simulink model "mc_sevcong4s10"  (R2025a)
settings: Solver=FixedStepAuto  StartTime=0.0  StopTime=10.0  FixedStep=0.05  RelTol=1e-3
settings Model: Creator=adam  LastModifiedBy=adam

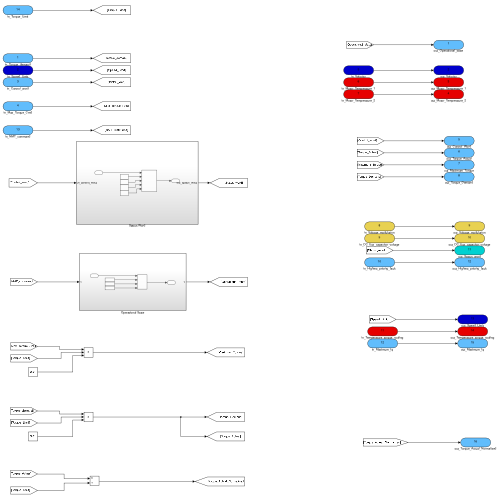
[thumbnail: Simulink's stored preview of the top-level diagram]
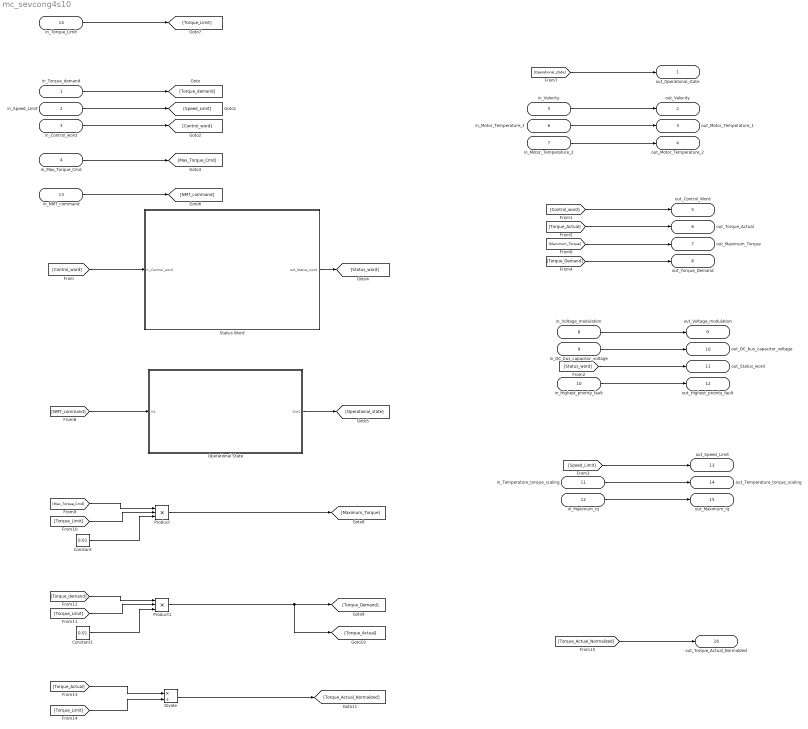
== system mc_sevcong4s10 ==
  in_Torque_demand : Inport
  in_Speed_Limit : Inport  Port=2
  in_Control_word : Inport  Port=3
  in_Max_Torque_Cmd : Inport  Port=4
  in_Velocity : Inport  Port=5
  in_Motor_Temperature_1 : Inport  Port=6
  in_Motor_Temperature_2 : Inport  Port=7
  in_Voltage_modulation : Inport  Port=8
  in_DC_bus_capacitor_voltage : Inport  Port=9
  in_Highest_priority_fault : Inport  Port=10
  in_Temperature_torque_scaling : Inport  Port=11
  in_Maximum_Iq : Inport  Port=12
  in_NMT_command : Inport  Port=13
  in_Torque_Limit : Inport  Port=14
  Constant : Constant  Value=0.01
  Constant1 : Constant  Value=0.01
  Divide : Product  Inputs=*/
  Operational State : Subsystem
  Product : Product  Inputs=3
  Product1 : Product  Inputs=3
  Status Word : Subsystem
  out_Operational_state : Outport
  out_Velocity : Outport  Port=2
  out_Motor_Temperature_1 : Outport  Port=3
  out_Motor_Temperature_2 : Outport  Port=4
  out_Control_Word : Outport  Port=5
  out_Torque_Actual : Outport  Port=6
  out_Maximum_Torque : Outport  Port=7
  out_Torque_Demand : Outport  Port=8
  out_Voltage_modulation : Outport  Port=9
  out_DC_bus_capacitor_voltage : Outport  Port=10
  out_Status_word : Outport  Port=11
  out_Highest_priority_fault : Outport  Port=12
  out_Speed_Limit : Outport  Port=13
  out_Temperature_torque_scaling : Outport  Port=14
  out_Maximum_Iq : Outport  Port=15
  out_Torque_Actual_Normalized : Outport  Port=16
  wires:
  in_Torque_demand/1 -> [Torque_demand]
  in_Speed_Limit/1 -> [Speed_Limit]
  in_Control_word/1 -> [Control_word]
  in_Max_Torque_Cmd/1 -> [Max_Torque_Cmd]
  in_Motor_Temperature_2/1 -> out_Motor_Temperature_2/1
  in_Velocity/1 -> out_Velocity/1
  in_Motor_Temperature_1/1 -> out_Motor_Temperature_1/1
  [Maximum_Torque] -> out_Maximum_Torque/1
  [Control_word] -> out_Control_Word/1
  [Torque_Demand] -> out_Torque_Demand/1
  in_DC_bus_capacitor_voltage/1 -> out_DC_bus_capacitor_voltage/1
  in_Voltage_modulation/1 -> out_Voltage_modulation/1
  [Status_word] -> out_Status_word/1
  in_Highest_priority_fault/1 -> out_Highest_priority_fault/1
  in_Maximum_Iq/1 -> out_Maximum_Iq/1
  in_Temperature_torque_scaling/1 -> out_Temperature_torque_scaling/1
  [Speed_Limit] -> out_Speed_Limit/1
  [Control_word] -> Status Word/1(in_Control_word)
  Status Word/1(out_Status_word) -> [Status_word]
  in_NMT_command/1 -> [NMT_command]
  [Operational_state] -> out_Operational_state/1
  in_Torque_Limit/1 -> [Torque_Limit]
  [NMT_command] -> Operational State/1(In1)
  Operational State/1(Out1) -> [Operational_state]
  [Torque_Actual] -> out_Torque_Actual/1
  [Max_Torque_Cmd] -> Product/1
  [Torque_Limit] -> Product/2
  Constant/1 -> Product/3
  Product/1 -> [Maximum_Torque]
  Product1/1 -> [Torque_Actual], [Torque_Demand]
  Constant1/1 -> Product1/3
  [Torque_Limit] -> Product1/2
  [Torque_demand] -> Product1/1
  [Torque_Actual] -> Divide/1
  [Torque_Limit] -> Divide/2
  Divide/1 -> [Torque_Actual_Normalized]
  [Torque_Actual_Normalized] -> out_Torque_Actual_Normalized/1

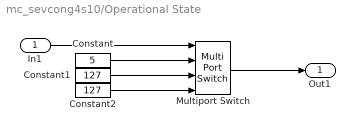
== system mc_sevcong4s10/Operational State ==
  In1 : Inport
  Constant : Constant  Value=5
  Constant1 : Constant  Value=127
  Constant2 : Constant  Value=127
  Multiport Switch : MultiPortSwitch  DataPortOrder=Specify indices  DataPortIndices={1,128}  DataPortForDefault=Additional data port  SaturateOnIntegerOverflow=off  InputSameDT=off
  Out1 : Outport
  wires:
  In1/1 -> Multiport Switch/1
  Multiport Switch/1 -> Out1/1
  Constant/1 -> Multiport Switch/2
  Constant2/1 -> Multiport Switch/4
  Constant1/1 -> Multiport Switch/3

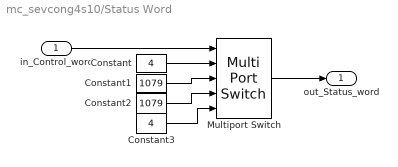
== system mc_sevcong4s10/Status Word ==
  in_Control_word : Inport
  Constant : Constant  Value=4
  Constant1 : Constant  Value=1079
  Constant2 : Constant  Value=1079
  Constant3 : Constant  Value=4
  Multiport Switch : MultiPortSwitch  DataPortOrder=Specify indices  DataPortIndices={6,7,15}  DataPortForDefault=Additional data port  DiagnosticForDefault=None  SaturateOnIntegerOverflow=off  InputSameDT=off
  out_Status_word : Outport
  wires:
  Multiport Switch/1 -> out_Status_word/1
  Constant/1 -> Multiport Switch/2
  Constant1/1 -> Multiport Switch/3
  Constant2/1 -> Multiport Switch/4
  Constant3/1 -> Multiport Switch/5
  in_Control_word/1 -> Multiport Switch/1
